simulink model "GNC_integrated_v4"  (R2023a)
settings: Solver=ode4  StartTime=0.0  StopTime=200  FixedStep=0.001  RelTol=1e-3
values from neighbouring files (symbols this model uses):
  baseMission = 1    [uavPackageDeliveryDataDict.sldd]
undefined symbols (not defined in the file or in its folder): param
libraries: simulink_extras x6, uavalgslib x4, simulink x2, robotcorelib x1, uavutilslib x1
settings Model: Creator=timme  LastModifiedBy=jipva
settings DebuggingCC: ParameterPrecisionLossMsg=none

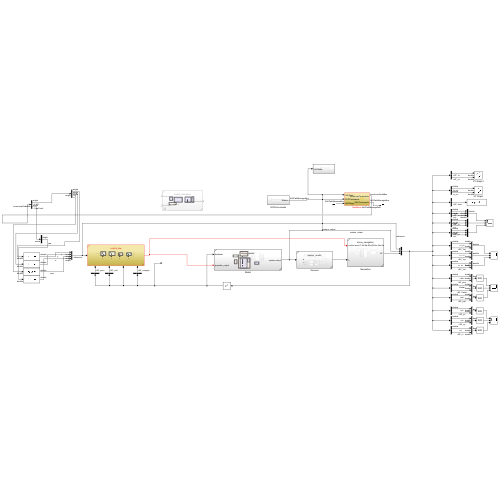
[thumbnail: Simulink's stored preview of the top-level diagram]
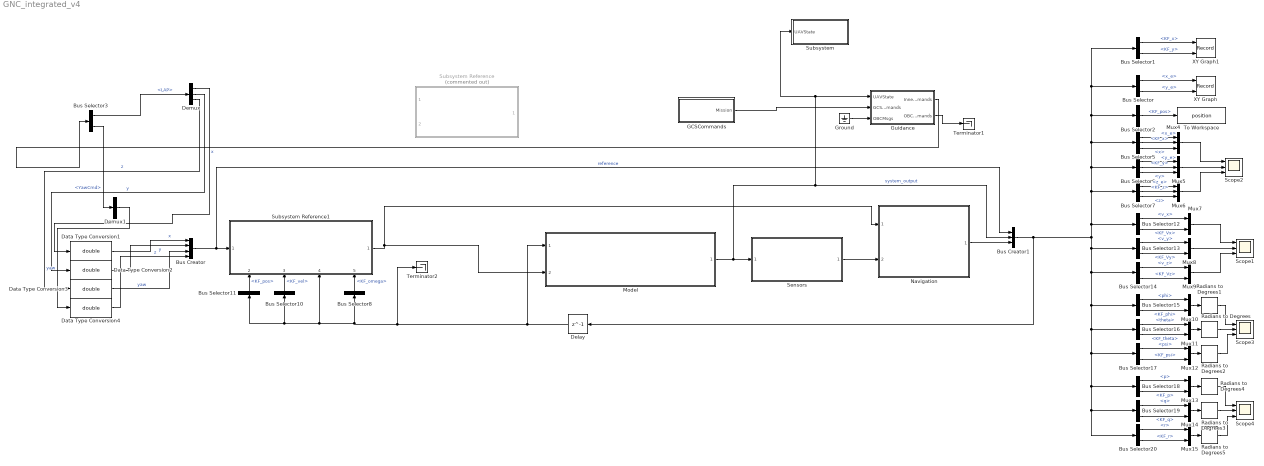
== system GNC_integrated_v4 ==
  Bus Creator : BusCreator  Inputs=4
  Bus Creator1 : BusCreator  Inputs=3
  Bus Selector : BusSelector  OutputSignals=system_output.pos.x_e,system_output.pos.y_e
  Bus Selector1 : BusSelector  OutputSignals=x_filt.KF_pos.KF_x,x_filt.KF_pos.KF_y
  Bus Selector10 : BusSelector  OutputSignals=x_filt.KF_vel
  Bus Selector11 : BusSelector  OutputSignals=x_filt.KF_pos
  Bus Selector12 : BusSelector  OutputSignals=system_output.V_e.v_x,x_filt.KF_vel.KF_Vx
  Bus Selector13 : BusSelector  OutputSignals=system_output.V_e.v_y,x_filt.KF_vel.KF_Vy
  Bus Selector14 : BusSelector  OutputSignals=system_output.V_e.v_z,x_filt.KF_vel.KF_Vz
  Bus Selector15 : BusSelector  OutputSignals=system_output.Att.phi,x_filt.KF_att.KF_phi
  Bus Selector16 : BusSelector  OutputSignals=system_output.Att.theta,x_filt.KF_att.KF_theta
  Bus Selector17 : BusSelector  OutputSignals=system_output.Att.psi,x_filt.KF_att.KF_psi
  Bus Selector18 : BusSelector  OutputSignals=system_output.ang_vel.p,x_filt.KF_omega.KF_p
  Bus Selector19 : BusSelector  OutputSignals=system_output.ang_vel.q,x_filt.KF_omega.KF_q
  Bus Selector2 : BusSelector  OutputSignals=x_filt.KF_pos
  Bus Selector20 : BusSelector  OutputSignals=system_output.ang_vel.r,x_filt.KF_omega.KF_r
  Bus Selector3 : BusSelector  OutputSignals=LAP,YawCmd
  Bus Selector5 : BusSelector  OutputSignals=system_output.pos.x_e,x_filt.KF_pos.KF_x,reference.x
  Bus Selector6 : BusSelector  OutputSignals=system_output.pos.y_e,x_filt.KF_pos.KF_y,reference.y
  Bus Selector7 : BusSelector  OutputSignals=system_output.pos.z_e,x_filt.KF_pos.KF_z,reference.z
  Bus Selector8 : BusSelector  OutputSignals=x_filt.KF_omega
  Data Type Conversion{1..4} (4 alike) : DataTypeConversion  OutDataTypeStr=double  SaturateOnIntegerOverflow=off  RndMeth=Floor
  Delay : Delay  DelayLength=1
  Demux : Demux  Outputs=3
  Demux1 : Demux  Outputs=1
  GCSCommands : Subsystem
  Ground : Ground
  Guidance : Subsystem
  Model : Subsystem  ReferencedSubsystem=drone_model
  Mux{7..15} (9 alike) : Mux  Inputs=2
  Mux4 : Mux  Inputs=3
  Mux5 : Mux  Inputs=3
  Mux6 : Mux  Inputs=3
  Navigation : Subsystem  ReferencedSubsystem=drone_navigation
  Radians to Degrees{,1..5} (6 alike) : simulink_extras/Transformations/Radians to Degrees
  Scope{1..4} (4 alike) : Scope  NumInputPorts=3
  Sensors : Subsystem  ReferencedSubsystem=sensor_model
  Subsystem : Subsystem
  Subsystem Reference : Subsystem  Commented=on  ReferencedSubsystem=control_allocation
  Subsystem Reference1 : Subsystem  ReferencedSubsystem=control_law
      settings: PortSchema="{\"entries\":[{\"content\":{\"sides\":[{\"content\":{\"connectorIds\":[\"In1\"]},\"type\":\"ConnectorPlacement.EquallySpacedRectSide\",\"uuid\":\"cbb659e7-d19a-4e68-9ae7-e5e39426296b\"},{\"content\":{\"connectorIds\":[\"Out1\"],\"side\":\"RIGHT\"},\"type\":\"ConnectorPlacement.EquallySpacedRectSide\",\"uuid\":\"c9f08a4e-80d9-41bf-93e6-4cfd11b32426\"},{\"content\":{\"side\":\"TOP\"},\"type\":\"ConnectorPlacement.EquallySpacedRectSide\",\"uuid\":\"8eafc22d-128e-4ca7-9eba-2c3fd299252c\"},{\"content\":{\"connectorIds\":[\"In2\",\"In3\",\"In4\",\"In5\"],\"side\":\"BOTTOM\"},\"type\":\"ConnectorPlacement.EquallySpacedRectSide\",\"uuid\":\"abe1dc09-e6b8-433e-beaf-ba54ebcb4b47\"}]},\"type\":\"ConnectorPlacement.EquallySpacedConnector\",\"uuid\":\"085ffc95-65e8-4235-be8d-72c324b16b8b\"}],\"packageUris\":[\"http://schema.mathworks.com/mf0/Connector/R2020b\"],\"version\":\"1.0\"}"
  Terminator1 : Terminator
  Terminator2 : Terminator
  To Workspace : ToWorkspace  VariableName=position  SaveFormat=Timeseries  SampleTime=param.dt
  XY Graph : Record  FileSettingsInternal="{\"entries\":[{\"content\":{\"excelSettings\":{\"content\":{},\"type\":\"Streamout.ExcelSettings\"}},\"type\":\"Streamout.FileSettingStorage\",\"uuid\":\"\"}],\"packageUris\":[\"http:\\/\\/schema.mathworks.com\\/mf0\\/streamout_blocks\\/R2020a\"],\"version\":\"1.0\"}"  Layout=[1 1]  SignalsInternal="{\"entries\":[{\"content\":{\"signals\":[{\"content\":{\"blockPath\":[],\"dimensions\":[1],\"domain\":\"\",\"lineColor\":\"#fe330a\",\"port\":1,\"sid\":[\"\"],\"signalID\":833,\"signalName\":\"<x_e>\"},\"type\":\"RecordBlkView.Signal\",\"uuid\":\"\"},{\"content\":{\"blockPath\":[],\"dimensions\":[1],\"domain\":\"\",\"lineColor\":\"#22b573\",\"port\":2,\"sid\":[\"\"],\"signalID\":837,\"signalName\":\"<y_e>\"},\"type\":\"RecordBlkView.Signal\",\"uuid\":\"\"}]},\"type\":\"RecordBlkView.InputSignals\",\"uuid\":\"\"}],\"packageUris\":[\"http:\\/\\/schema.mathworks.com\\/mf0\\/streamout_blocks\\/R2020a\"],\"version\":\"1.0\"}"  VisualizationBindings="{\"xyplotplugin\":{\"info\":[{\"series\":[],\"subplotID\":1}]}}"  CompatibilityTag=XY
  XY Graph1 : Record  FileSettingsInternal="{\"entries\":[{\"content\":{\"excelSettings\":{\"content\":{},\"type\":\"Streamout.ExcelSettings\"}},\"type\":\"Streamout.FileSettingStorage\",\"uuid\":\"\"}],\"packageUris\":[\"http:\\/\\/schema.mathworks.com\\/mf0\\/streamout_blocks\\/R2020a\"],\"version\":\"1.0\"}"  Layout=[1 1]  SignalsInternal="{\"entries\":[{\"content\":{\"signals\":[{\"content\":{\"blockPath\":[],\"dimensions\":[1],\"domain\":\"\",\"lineColor\":\"#0072bd\",\"port\":1,\"sid\":[\"\"],\"signalID\":841,\"signalName\":\"<KF_x>\"},\"type\":\"RecordBlkView.Signal\",\"uuid\":\"\"},{\"content\":{\"blockPath\":[],\"dimensions\":[1],\"domain\":\"\",\"lineColor\":\"#d95319\",\"port\":2,\"sid\":[\"\"],\"signalID\":845,\"signalName\":\"<KF_y>\"},\"type\":\"RecordBlkView.Signal\",\"uuid\":\"\"}]},\"type\":\"RecordBlkView.InputSignals\",\"uuid\":\"\"}],\"packageUris\":[\"http:\\/\\/schema.mathworks.com\\/mf0\\/streamout_blocks\\/R2020a\"],\"version\":\"1.0\"}"  VisualizationBindings="{\"xyplotplugin\":{\"info\":[{\"series\":[],\"subplotID\":1}]}}"  CompatibilityTag=XY
  wires:
  Bus Selector5/1 -> Mux4/1  "<x_e>"
  Bus Selector5/2 -> Mux4/2  "<KF_x>"
  Bus Selector6/1 -> Mux5/1  "<y_e>"
  Bus Selector6/2 -> Mux5/2  "<KF_y>"
  Bus Selector7/2 -> Mux6/2  "<KF_z>"
  Bus Selector7/1 -> Mux6/1  "<z_e>"
  Bus Selector12/2 -> Mux7/2  "<KF_Vx>"
  Bus Selector12/1 -> Mux7/1  "<v_x>"
  Bus Selector13/1 -> Mux8/1  "<v_y>"
  Bus Selector14/2 -> Mux9/2  "<KF_Vz>"
  Bus Selector14/1 -> Mux9/1  "<v_z>"
  Bus Selector13/2 -> Mux8/2  "<KF_Vy>"
  Bus Selector16/2 -> Mux11/2  "<KF_theta>"
  Mux12/1 -> Radians to Degrees2/1
  Mux11/1 -> Radians to Degrees/1
  Bus Selector17/2 -> Mux12/2  "<KF_psi>"
  Bus Selector17/1 -> Mux12/1  "<psi>"
  Bus Selector15/2 -> Mux10/2  "<KF_phi>"
  Mux10/1 -> Radians to Degrees1/1
  Bus Selector15/1 -> Mux10/1  "<phi>"
  Bus Selector16/1 -> Mux11/1  "<theta>"
  Bus Selector19/2 -> Mux14/2  "<KF_q>"
  Bus Selector18/2 -> Mux13/2  "<KF_p>"
  Mux13/1 -> Radians to Degrees4/1
  Bus Selector20/1 -> Mux15/1  "<r>"
  Bus Selector18/1 -> Mux13/1  "<p>"
  Mux15/1 -> Radians to Degrees5/1
  Bus Selector20/2 -> Mux15/2  "<KF_r>"
  Mux14/1 -> Radians to Degrees3/1
  Bus Selector19/1 -> Mux14/1  "<q>"
  Bus Selector/1 -> XY Graph/1  "<x_e>"
  Bus Selector/2 -> XY Graph/2  "<y_e>"
  Mux5/1 -> Scope2/2
  Mux4/1 -> Scope2/1
  Mux6/1 -> Scope2/3
  Mux8/1 -> Scope1/2
  Mux9/1 -> Scope1/3
  Mux7/1 -> Scope1/1
  Radians to Degrees2/1 -> Scope3/3
  Radians to Degrees1/1 -> Scope3/1
  Radians to Degrees/1 -> Scope3/2
  Radians to Degrees5/1 -> Scope4/3
  Radians to Degrees4/1 -> Scope4/1
  Radians to Degrees3/1 -> Scope4/2
  Bus Selector1/1 -> XY Graph1/1  "<KF_x>"
  Bus Selector1/2 -> XY Graph1/2  "<KF_y>"
  Sensors/1 -> Navigation/2
  Navigation/1 -> Bus Creator1/3
  Bus Selector2/1 -> To Workspace/1  "<KF_pos>"
  Bus Creator1/1 -> Delay/1, Bus Selector13/1, Bus Selector14/1, Bus Selector20/1, Bus Selector19/1, Bus Selector18/1, Bus Selector17/1, Bus Selector16/1, Bus Selector15/1, Bus Selector12/1, Bus Selector7/1, Bus Selector6/1, Bus Selector2/1, Bus Selector1/1, Bus Selector/1, Bus Selector5/1
  Bus Creator/1 -> Bus Creator1/1, Subsystem Reference1/1  "reference"
  Bus Selector11/1 -> Subsystem Reference1/2  "<KF_pos>"
  Bus Selector10/1 -> Subsystem Reference1/3  "<KF_vel>"
  Delay/1 -> Model/1, Terminator2/1, Bus Selector8/1, Subsystem Reference1/4, Bus Selector11/1, Bus Selector10/1
  Bus Selector8/1 -> Subsystem Reference1/5  "<KF_omega>"
  Bus Selector5/3 -> Mux4/3  "<x>"
  Bus Selector6/3 -> Mux5/3  "<y>"
  Bus Selector7/3 -> Mux6/3  "<z>"
  Subsystem Reference1/1 -> Model/2, Navigation/1
  GCSCommands/1(Mission) -> Guidance/2(GCSCommands)
  Guidance/2(OBCCommands) -> Terminator1/1
  Model/1 -> Sensors/1, Guidance/1(UAVState), Subsystem/1(UAVState), Bus Creator1/2  "system_output"
  Ground/1 -> Guidance/3(OBCMsgs)
  Bus Selector3/1 -> Demux/1  "<LAP>"
  Demux/1 -> Data Type Conversion1/1  "x"
  Demux/2 -> Data Type Conversion2/1  "y"
  Demux/3 -> Data Type Conversion3/1  "z"
  Bus Selector3/2 -> Demux1/1  "<YawCmd>"
  Demux1/1 -> Data Type Conversion4/1  "yaw"
  Guidance/1(InnerLoopCommands) -> Bus Selector3/1
  Data Type Conversion1/1 -> Bus Creator/1  "x"
  Data Type Conversion2/1 -> Bus Creator/2  "y"
  Data Type Conversion3/1 -> Bus Creator/3  "yaw"
  Data Type Conversion4/1 -> Bus Creator/4  "z"

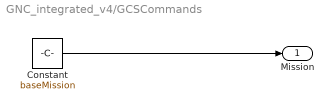
== system GNC_integrated_v4/GCSCommands ==
  Constant : Constant  Value=baseMission  OutDataTypeStr=Bus: UAVPathManagerBus  SampleTime=-1
  Mission : Outport
  wires:
  Constant/1 -> Mission/1

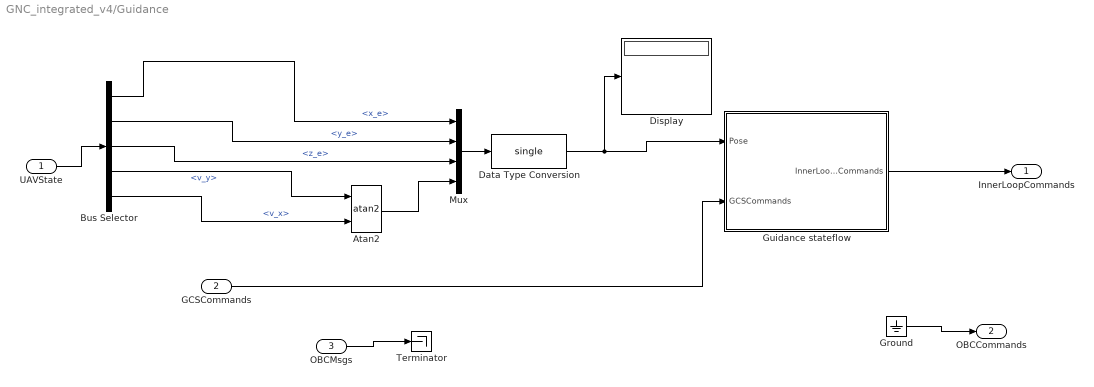
== system GNC_integrated_v4/Guidance ==
  UAVState : Inport
  GCSCommands : Inport  Port=2
  OBCMsgs : Inport  Port=3
  Atan2 : Trigonometry  Operator=atan2
  Bus Selector : BusSelector  OutputSignals=pos.x_e,pos.y_e,pos.z_e,V_e.v_y,V_e.v_x
  Data Type Conversion : DataTypeConversion  OutDataTypeStr=single  SaturateOnIntegerOverflow=off  RndMeth=Floor
  Display : Display
  Ground : Ground
  Guidance stateflow : Subsystem
  Mux : Mux
  Terminator : Terminator
  InnerLoopCommands : Outport
  OBCCommands : Outport  Port=2  OutDataTypeStr=Bus: UAVPathManagerBus
  wires:
  Atan2/1 -> Mux/4
  GCSCommands/1 -> Guidance stateflow/2(GCSCommands)
  OBCMsgs/1 -> Terminator/1
  Guidance stateflow/1(InnerLoopCommands) -> InnerLoopCommands/1
  Ground/1 -> OBCCommands/1
  UAVState/1 -> Bus Selector/1
  Bus Selector/1 -> Mux/1  "<x_e>"
  Bus Selector/2 -> Mux/2  "<y_e>"
  Bus Selector/3 -> Mux/3  "<z_e>"
  Bus Selector/4 -> Atan2/1  "<v_y>"
  Bus Selector/5 -> Atan2/2  "<v_x>"
  Mux/1 -> Data Type Conversion/1
  Data Type Conversion/1 -> Display/1, Guidance stateflow/1(Pose)

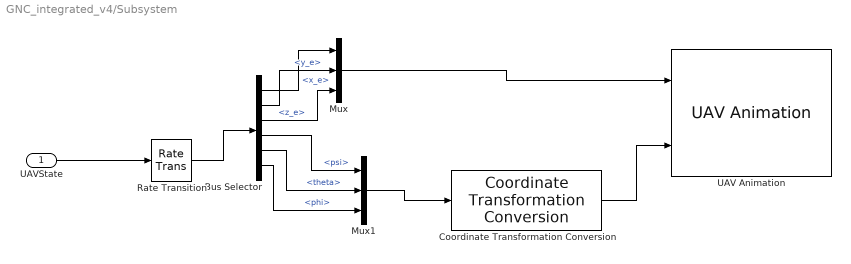
== system GNC_integrated_v4/Subsystem ==
  UAVState : Inport
  Bus Selector : BusSelector  OutputSignals=pos.x_e,pos.y_e,pos.z_e,Att.psi,Att.theta,Att.phi
  Coordinate Transformation Conversion : robotcorelib/Coordinate Transformation Conversion  InputRepresentation=Euler Angles  InputEulerSequence=ZYX  ShowTrVecInputPort=on  OutputRepresentation=Quaternion  OutputEulerSequence=ZYX  ShowTrVecOutputPort=on  SimulateUsing=Code generation
      settings: LibrarySourceBlock=navlib/Utilities/Coordinate Transformation Conversion
  Mux : Mux  Inputs=3
  Mux1 : Mux  Inputs=3
  Rate Transition : RateTransition  OutPortSampleTime=1
  UAV Animation : uavutilslib/UAV Animation  UAVType=Multirotor  UAVSize=1  InertialZDirection=Down  SampleTime=-1
  wires:
  UAVState/1 -> Rate Transition/1
  Rate Transition/1 -> Bus Selector/1
  Bus Selector/1 -> Mux/1  "<x_e>"
  Bus Selector/2 -> Mux/2  "<y_e>"
  Bus Selector/3 -> Mux/3  "<z_e>"
  Bus Selector/4 -> Mux1/1  "<psi>"
  Bus Selector/5 -> Mux1/2  "<theta>"
  Bus Selector/6 -> Mux1/3  "<phi>"
  Mux1/1 -> Coordinate Transformation Conversion/1
  Coordinate Transformation Conversion/1 -> UAV Animation/2
  Mux/1 -> UAV Animation/1

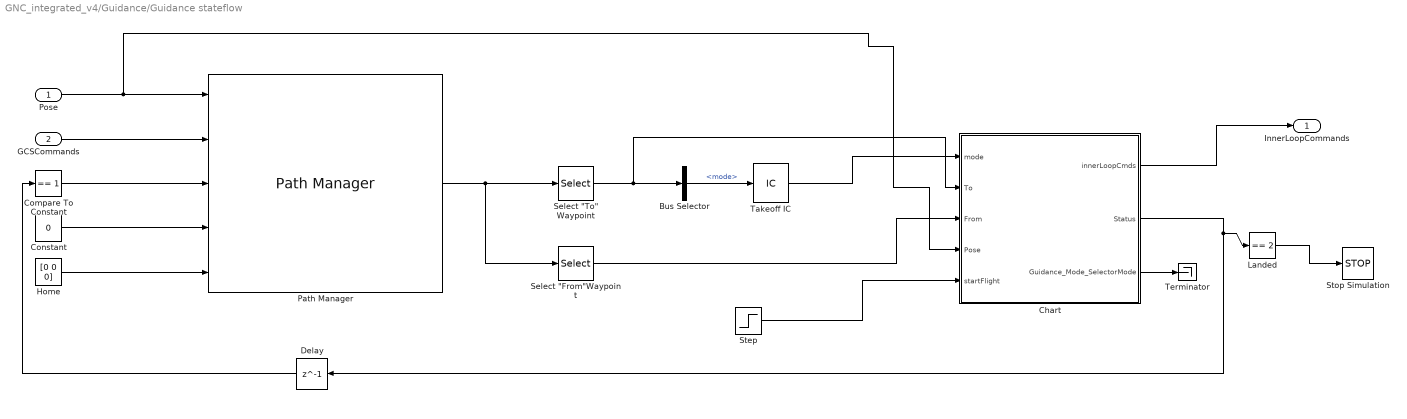
== system GNC_integrated_v4/Guidance/Guidance stateflow ==
  Pose : Inport
  GCSCommands : Inport  Port=2
  Bus Selector : BusSelector  OutputSignals=mode
  Chart : Stateflow chart  TreatAsAtomicUnit=on
  Compare To Constant : simulink/Logic and Bit Operations/Compare To Constant  relop===  const=1  OutDataTypeStr=boolean
  Constant : Constant  Value=0  OutDataTypeStr=uint8
  Delay : Delay  DelayLength=1  InitialCondition=0
  Home : Constant  Value=[0 0 0]  OutDataTypeStr=single
  Landed : simulink/Logic and Bit Operations/Compare To Constant  relop===  const=2  OutDataTypeStr=boolean
  Path Manager : uavalgslib/Path Manager  UAVType=multirotor  LoiterRadius=25  dataType=single  inputBusName='UAVPathManagerBus'  SimulateUsing=Code generation
  "Select \"From\"Waypoint" : Selector  InputPortWidth=2  IndexOptions=Index vector (dialog)  Indices=2  OutputSizes=1
  "Select \"To\" Waypoint" : Selector  InputPortWidth=2  IndexOptions=Index vector (dialog)  Indices=1  OutputSizes=1
  Step : Step  Time=0.5  SampleTime=0.02
  Stop Simulation : Stop
  Takeoff IC : InitialCondition
  Terminator : Terminator
  InnerLoopCommands : Outport  OutDataTypeStr=Bus: innerLoopCmdsBus
  wires:
  GCSCommands/1 -> Path Manager/2
  Home/1 -> Path Manager/5
  Constant/1 -> Path Manager/4
  Path Manager/1 -> "Select \"From\"Waypoint"/1, "Select \"To\" Waypoint"/1
  Bus Selector/1 -> Takeoff IC/1  "<mode>"
  Delay/1 -> Compare To Constant/1
  Compare To Constant/1 -> Path Manager/3
  Step/1 -> Chart/5(startFlight)
  Landed/1 -> Stop Simulation/1
  Pose/1 -> Chart/4(Pose), Path Manager/1
  "Select \"To\" Waypoint"/1 -> Chart/2(To), Bus Selector/1
  "Select \"From\"Waypoint"/1 -> Chart/3(From)
  Chart/1(innerLoopCmds) -> InnerLoopCommands/1
  Chart/2(Status) -> Delay/1, Landed/1
  Takeoff IC/1 -> Chart/1(mode)
  Chart/3(Guidance_Mode_SelectorMode) -> Terminator/1

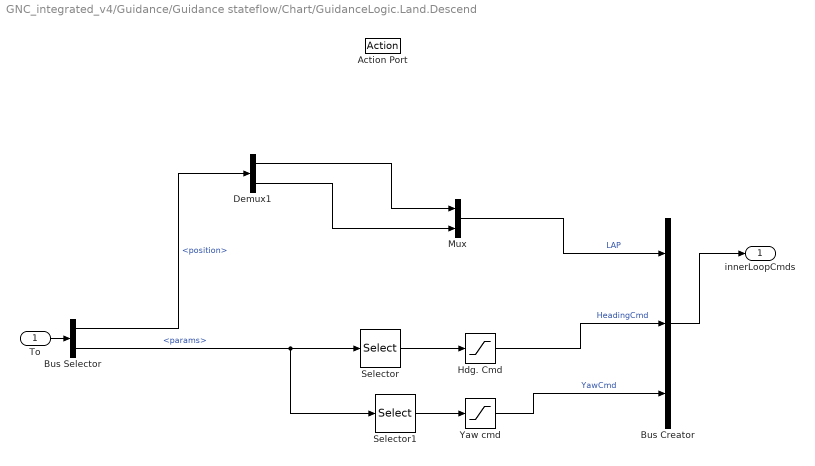
== system GNC_integrated_v4/Guidance/Guidance stateflow/Chart/GuidanceLogic.Land.Descend ==
  To : Inport
  Action Port : ActionPort
      settings: CopyFcn=Stateflow.SLINSF.SimulinkMan.removeBlockPreDeleteFcn  PreDeleteFcn=Stateflow.SLINSF.SimulinkMan.unsafePredeleteFcn
  Bus Creator : BusCreator  Inputs=3  OutDataTypeStr=Bus: innerLoopCmdsBus  NonVirtualBus=on
  Bus Selector : BusSelector  OutputSignals=position,params
  Demux1 : Demux  Outputs=[2 1]
  Hdg. Cmd : Saturate
  Mux : Mux  Inputs=2
  Selector : Selector  InputPortWidth=4  IndexOptions=Index vector (dialog)  Indices=4  OutputSizes=1
  Selector1 : Selector  InputPortWidth=4  IndexOptions=Index vector (dialog)  Indices=4  OutputSizes=1
  Yaw cmd : Saturate  UpperLimit=pi  LowerLimit=-pi
  innerLoopCmds : Outport  OutDataTypeStr=Bus: innerLoopCmdsBus
  wires:
  Bus Selector/1 -> Demux1/1  "<position>"
  Demux1/2 -> Mux/2
  Mux/1 -> Bus Creator/1  "LAP"
  Bus Selector/2 -> Selector1/1, Selector/1  "<params>"
  Selector1/1 -> Yaw cmd/1
  Demux1/1 -> Mux/1
  Hdg. Cmd/1 -> Bus Creator/2  "HeadingCmd"
  Selector/1 -> Hdg. Cmd/1
  Yaw cmd/1 -> Bus Creator/3  "YawCmd"
  Bus Creator/1 -> innerLoopCmds/1
  To/1 -> Bus Selector/1

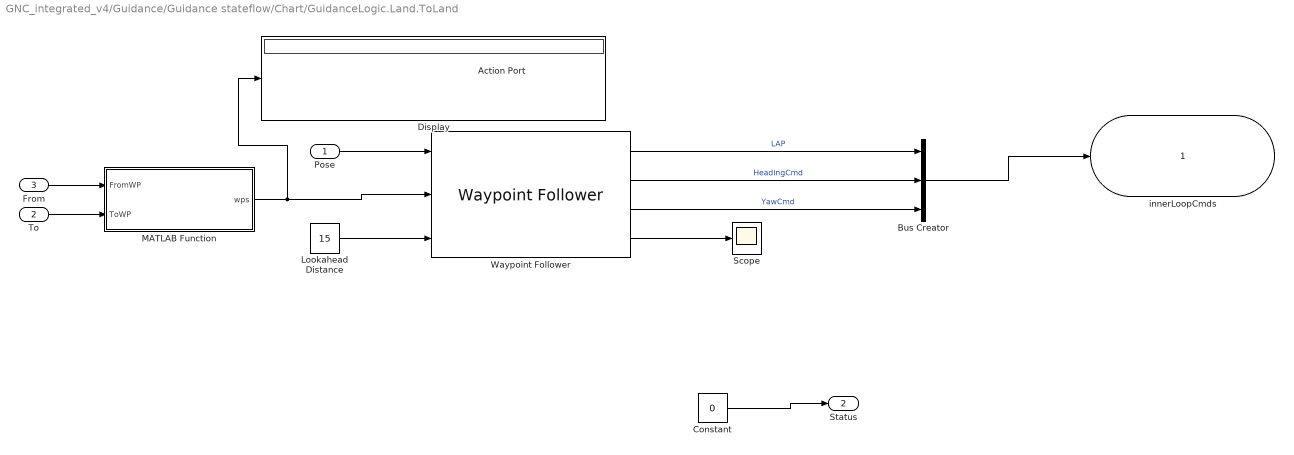
== system GNC_integrated_v4/Guidance/Guidance stateflow/Chart/GuidanceLogic.Land.ToLand ==
  Pose : Inport
  To : Inport  Port=2
  From : Inport  Port=3
  Action Port : ActionPort
      settings: CopyFcn=Stateflow.SLINSF.SimulinkMan.removeBlockPreDeleteFcn  PreDeleteFcn=Stateflow.SLINSF.SimulinkMan.unsafePredeleteFcn
  Bus Creator : BusCreator  Inputs=3  OutDataTypeStr=Bus: innerLoopCmdsBus  NonVirtualBus=on
  Constant : Constant  Value=0  OutDataTypeStr=uint8
  Display : Display
  Lookahead Distance : Constant  Value=15  OutDataTypeStr=single
  MATLAB Function : MATLAB Function  TreatAsAtomicUnit=on
  Scope : Scope
  Waypoint Follower : uavalgslib/Waypoint Follower  UAVType=multirotor  StartFrom=first  TransitionRadiusSource=internal  TransitionRadius=10  MinLookaheadDistance=0.1  YawInput=on  ShowCrossTrackErrorOutput=off  ShowStatusOutput=off  SimulateUsing=Interpreted execution
  innerLoopCmds : Outport  OutDataTypeStr=Bus: innerLoopCmdsBus
  Status : Outport  Port=2
  wires:
  To/1 -> MATLAB Function/2(ToWP)
  MATLAB Function/1(wps) -> Display/1, Waypoint Follower/2
  Waypoint Follower/1 -> Bus Creator/1  "LAP"
  Bus Creator/1 -> innerLoopCmds/1
  From/1 -> MATLAB Function/1(FromWP)
  Pose/1 -> Waypoint Follower/1
  Waypoint Follower/2 -> Bus Creator/2  "HeadingCmd"
  Waypoint Follower/4 -> Scope/1
  Lookahead Distance/1 -> Waypoint Follower/3
  Waypoint Follower/3 -> Bus Creator/3  "YawCmd"
  Constant/1 -> Status/1

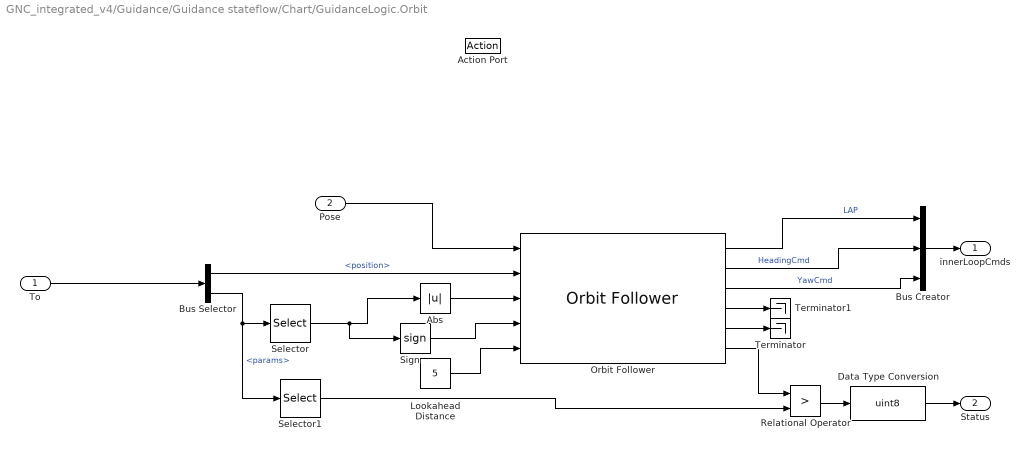
== system GNC_integrated_v4/Guidance/Guidance stateflow/Chart/GuidanceLogic.Orbit ==
  To : Inport
  Pose : Inport  Port=2
  Action Port : ActionPort
      settings: CopyFcn=Stateflow.SLINSF.SimulinkMan.removeBlockPreDeleteFcn  PreDeleteFcn=Stateflow.SLINSF.SimulinkMan.unsafePredeleteFcn
  Abs : Abs  SaturateOnIntegerOverflow=off
  Bus Creator : BusCreator  Inputs=3  OutDataTypeStr=Bus: innerLoopCmdsBus  NonVirtualBus=on
  Bus Selector : BusSelector  OutputSignals=position,params
  Data Type Conversion : DataTypeConversion  OutDataTypeStr=uint8  SaturateOnIntegerOverflow=off  RndMeth=Floor
  Lookahead Distance : Constant  Value=5  OutDataTypeStr=single
  Orbit Follower : uavalgslib/Orbit Follower  UAVType=multirotor  MinOrbitRadius=1  MinLookaheadDistance=0.1  ExternalReset=none  ShowCrossTrackErrorOutput=off  ShowNumTurnsOutput=on  SimulateUsing=Code generation
  Relational Operator : RelationalOperator  Operator=>  OutDataTypeStr=boolean  RndMeth=Simplest  InputSameDT=off
  Selector : Selector  InputPortWidth=4  IndexOptions=Index vector (dialog)  Indices=[3]  OutputSizes=1
  Selector1 : Selector  InputPortWidth=4  IndexOptions=Index vector (dialog)  Indices=[1]  OutputSizes=1
  Sign : Signum
  Terminator : Terminator
  Terminator1 : Terminator
  innerLoopCmds : Outport  OutDataTypeStr=Bus: innerLoopCmdsBus
  Status : Outport  Port=2
  wires:
  To/1 -> Bus Selector/1
  Orbit Follower/4 -> Terminator1/1
  Orbit Follower/5 -> Terminator/1
  Orbit Follower/1 -> Bus Creator/1  "LAP"
  Orbit Follower/2 -> Bus Creator/2  "HeadingCmd"
  Orbit Follower/3 -> Bus Creator/3  "YawCmd"
  Bus Creator/1 -> innerLoopCmds/1
  Pose/1 -> Orbit Follower/1
  Bus Selector/1 -> Orbit Follower/2  "<position>"
  Bus Selector/2 -> Selector1/1, Selector/1  "<params>"
  Abs/1 -> Orbit Follower/3
  Selector/1 -> Sign/1, Abs/1
  Lookahead Distance/1 -> Orbit Follower/5
  Sign/1 -> Orbit Follower/4
  Orbit Follower/6 -> Relational Operator/1
  Selector1/1 -> Relational Operator/2
  Relational Operator/1 -> Data Type Conversion/1
  Data Type Conversion/1 -> Status/1

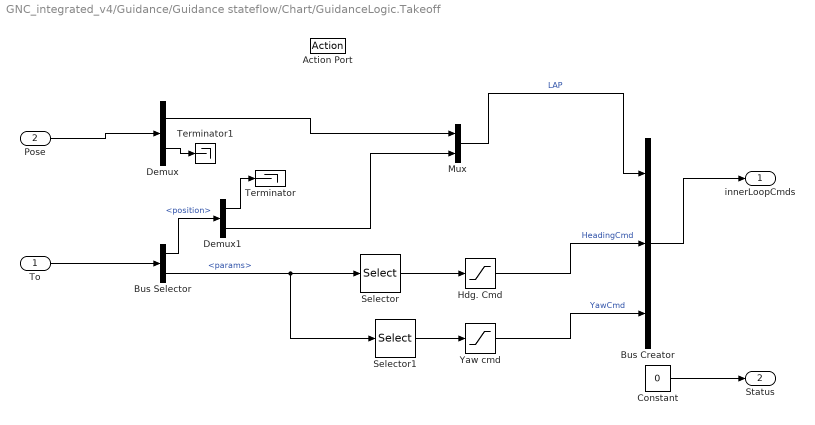
== system GNC_integrated_v4/Guidance/Guidance stateflow/Chart/GuidanceLogic.Takeoff ==
  To : Inport
  Pose : Inport  Port=2
  Action Port : ActionPort
      settings: CopyFcn=Stateflow.SLINSF.SimulinkMan.removeBlockPreDeleteFcn  PreDeleteFcn=Stateflow.SLINSF.SimulinkMan.unsafePredeleteFcn
  Bus Creator : BusCreator  Inputs=3  OutDataTypeStr=Bus: innerLoopCmdsBus  NonVirtualBus=on
  Bus Selector : BusSelector  OutputSignals=position,params
  Constant : Constant  Value=0  OutDataTypeStr=uint8
  Demux : Demux  Outputs=[2 2]
  Demux1 : Demux  Outputs=2
  Hdg. Cmd : Saturate
  Mux : Mux  Inputs=2
  Selector : Selector  InputPortWidth=4  IndexOptions=Index vector (dialog)  Indices=4  OutputSizes=1
  Selector1 : Selector  InputPortWidth=4  IndexOptions=Index vector (dialog)  Indices=4  OutputSizes=1
  Terminator : Terminator
  Terminator1 : Terminator
  Yaw cmd : Saturate  UpperLimit=pi  LowerLimit=-pi
  innerLoopCmds : Outport  OutDataTypeStr=Bus: innerLoopCmdsBus
  Status : Outport  Port=2
  wires:
  Pose/1 -> Demux/1
  Demux/1 -> Mux/1
  Mux/1 -> Bus Creator/1  "LAP"
  To/1 -> Bus Selector/1
  Bus Selector/1 -> Demux1/1  "<position>"
  Demux1/1 -> Terminator/1
  Demux1/2 -> Mux/2
  Bus Selector/2 -> Selector1/1, Selector/1  "<params>"
  Bus Creator/1 -> innerLoopCmds/1
  Demux/2 -> Terminator1/1
  Hdg. Cmd/1 -> Bus Creator/2  "HeadingCmd"
  Selector1/1 -> Yaw cmd/1
  Selector/1 -> Hdg. Cmd/1
  Yaw cmd/1 -> Bus Creator/3  "YawCmd"
  Constant/1 -> Status/1

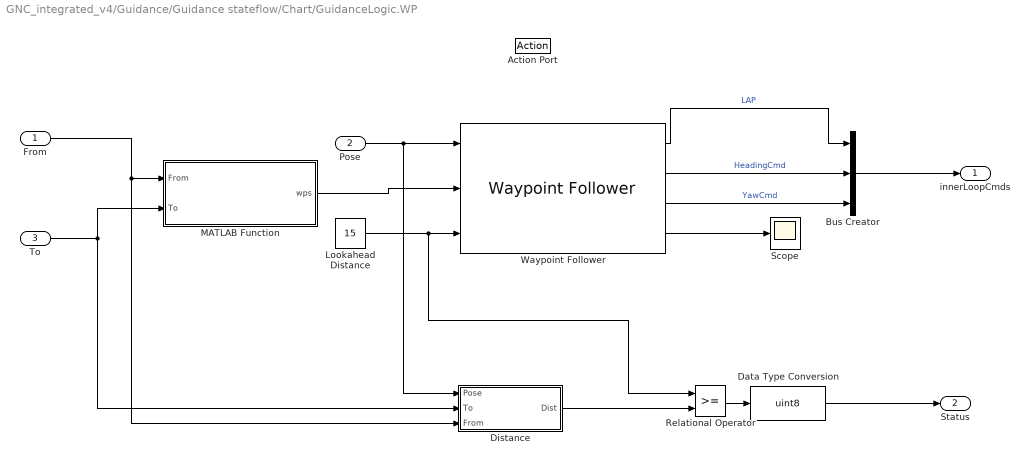
== system GNC_integrated_v4/Guidance/Guidance stateflow/Chart/GuidanceLogic.WP ==
  From : Inport
  Pose : Inport  Port=2
  To : Inport  Port=3
  Action Port : ActionPort
      settings: CopyFcn=Stateflow.SLINSF.SimulinkMan.removeBlockPreDeleteFcn  PreDeleteFcn=Stateflow.SLINSF.SimulinkMan.unsafePredeleteFcn
  Bus Creator : BusCreator  Inputs=3  OutDataTypeStr=Bus: innerLoopCmdsBus  NonVirtualBus=on
  Data Type Conversion : DataTypeConversion  OutDataTypeStr=uint8  SaturateOnIntegerOverflow=off  RndMeth=Floor
  Distance : Subsystem
  Lookahead Distance : Constant  Value=15  OutDataTypeStr=single
  MATLAB Function : MATLAB Function  TreatAsAtomicUnit=on
  Relational Operator : RelationalOperator  OutDataTypeStr=boolean  RndMeth=Simplest  InputSameDT=off
  Scope : Scope
  Waypoint Follower : uavalgslib/Waypoint Follower  UAVType=multirotor  StartFrom=first  TransitionRadiusSource=internal  TransitionRadius=10  MinLookaheadDistance=0.1  YawInput=off  ShowCrossTrackErrorOutput=off  ShowStatusOutput=off  SimulateUsing=Interpreted execution
  innerLoopCmds : Outport  OutDataTypeStr=Bus: innerLoopCmdsBus
  Status : Outport  Port=2
  wires:
  To/1 -> MATLAB Function/2(To), Distance/2(To)
  MATLAB Function/1(wps) -> Waypoint Follower/2
  Waypoint Follower/1 -> Bus Creator/1  "LAP"
  Data Type Conversion/1 -> Status/1
  Bus Creator/1 -> innerLoopCmds/1
  From/1 -> Distance/3(From), MATLAB Function/1(From)
  Pose/1 -> Distance/1(Pose), Waypoint Follower/1
  Waypoint Follower/2 -> Bus Creator/2  "HeadingCmd"
  Waypoint Follower/4 -> Scope/1
  Relational Operator/1 -> Data Type Conversion/1
  Distance/1(Dist) -> Relational Operator/2
  Lookahead Distance/1 -> Relational Operator/1, Waypoint Follower/3
  Waypoint Follower/3 -> Bus Creator/3  "YawCmd"

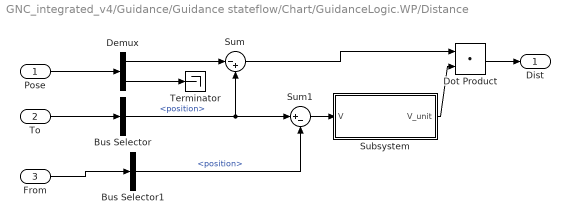
== system GNC_integrated_v4/Guidance/Guidance stateflow/Chart/GuidanceLogic.WP/Distance ==
  Pose : Inport
  To : Inport  Port=2
  From : Inport  Port=3
  Bus Selector : BusSelector  OutputSignals=position
  Bus Selector1 : BusSelector  OutputSignals=position
  Demux : Demux  Outputs=[3 1]
  Dot Product : DotProduct  OutDataTypeStr=Inherit: Inherit via internal rule
  Subsystem : Subsystem
  Sum : Sum  Inputs=|-+
  Sum1 : Sum  Inputs=|+-
  Terminator : Terminator
  Dist : Outport
  wires:
  Pose/1 -> Demux/1
  Demux/1 -> Sum/1
  Demux/2 -> Terminator/1
  To/1 -> Bus Selector/1
  From/1 -> Bus Selector1/1
  Bus Selector1/1 -> Sum1/2  "<position>"
  Bus Selector/1 -> Sum/2, Sum1/1  "<position>"
  Sum/1 -> Dot Product/1
  Dot Product/1 -> Dist/1
  Sum1/1 -> Subsystem/1(V)
  Subsystem/1(V_unit) -> Dot Product/2

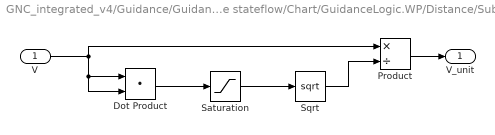
== system GNC_integrated_v4/Guidance/Guidance stateflow/Chart/GuidanceLogic.WP/Distance/Subsystem ==
  V : Inport
  Dot Product : DotProduct  OutDataTypeStr=Inherit: Inherit via internal rule
  Product : Product  Inputs=*/
  Saturation : Saturate
  Sqrt : Sqrt
  V_unit : Outport
  wires:
  Dot Product/1 -> Saturation/1
  Saturation/1 -> Sqrt/1
  V/1 -> Dot Product/1, Dot Product/2, Product/1
  Product/1 -> V_unit/1
  Sqrt/1 -> Product/2

== matlab function GNC_integrated_v4/Guidance/Guidance stateflow/Chart/GuidanceLogic.Land.ToLand/MATLAB Function ==
  data: FromWP input; wps output; ToWP input
function wps = getLandingWaypoint(FromWP, ToWP)

persistent outWPS

if isempty(outWPS)
    outWPS = single(zeros(2,4));
end

outWPS(1,:) = [FromWP.position' FromWP.params(4)];
outWPS(2,:) = [ToWP.position(1:2)' FromWP.position(3) ToWP.params(4)];

wps = outWPS;

== matlab function GNC_integrated_v4/Guidance/Guidance stateflow/Chart/GuidanceLogic.WP/MATLAB Function ==
  data: From input Bus: UAVPathManagerBus; wps output; To input Bus: UAVPathManagerBus
function wps = getWaypointMission(From, To)

persistent outWPS

if isempty(outWPS)
    outWPS = single(zeros(2,4));
end

outWPS(1,:) = [From.position' From.params(4)];
outWPS(2,:) = [To.position' To.params(4)];

% for ii=1:2
%     outWPS(ii,1:3) = GCSMission(ii).position';
%     outWPS(ii,4) = GCSMission(ii).params(4);
% end

wps = outWPS;

== stateflow chart GNC_integrated_v4/Guidance/Guidance stateflow/Chart ==
  settings: updateMethod=DISCRETE  sampleTime=0.02
  state GuidanceLogic
    state OnGround
    state Takeoff
    state WP
    state Orbit
    state Land
      state ToLand
      state Descend
      (default) -> ToLand
      ToLand -> Descend
    (default) -> OnGround
    OnGround -> (junction 12) : [startFlight == 1]
    GuidanceLogic -> (junction 12) : [hasChanged(mode)]
    (junction 12) -> Takeoff [order 1] : [Pose(3) >= 1]
    (junction 12) -> (junction 10) [order 2]
    Takeoff -> WP : [Pose(3) <= To.position(3)]{Status = 1;}
    (junction 10) -> WP [order 1] : [mode == 2]
    (junction 10) -> (junction 11) [order 2]
    (junction 11) -> Orbit [order 1] : [mode == 3]
    (junction 11) -> (junction 29) [order 2]
    (junction 29) -> Land
    Land -> GuidanceLogic : [Pose(3) >= -0.1]{Status = 2;}
  (default) -> GuidanceLogic
  data: sf_internal_action_state_placeholder_data local double size=1 =0; sf_internal_action_state_placeholder_data local double size=1 =0; sf_internal_action_state_placeholder_data local double size=1 =0; sf_internal_action_state_placeholder_data local double size=1 =0; sf_internal_action_state_placeholder_data local double size=1 =0; innerLoopCmds output Bus: innerLoopCmdsBus; Status output uint8; mode input; To input Bus: UAVPathManagerBus; From input Bus: UAVPathManagerBus; Pose input; startFlight input; Guidance_Mode_SelectorMode output Enum: Guidance_Mode_SelectorModeType
